simulink model "MODEL_R2021a"  (R2021a)
settings: Solver=FixedStepAuto  StartTime=0.0  StopTime=10.0  FixedStep=0.01  RelTol=1e-3
PreLoadFcn:
  | run('MAIN.m');
undefined symbols (not defined in the file or in its folder): d0, u0, u_tilde
settings Model: OrderedModelArguments=off  Creator=atavo  LastModifiedBy=atavo

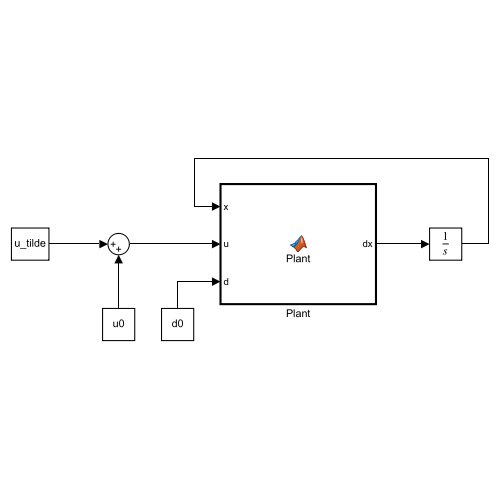
[thumbnail: Simulink's stored preview of the top-level diagram]
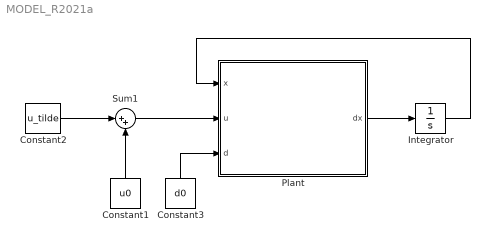
== system MODEL_R2021a ==
  Constant1 : Constant  Value=u0
  Constant2 : Constant  Value=u_tilde
  Constant3 : Constant  Value=d0
  Integrator : Integrator
  Plant : MATLAB Function  TreatAsAtomicUnit=on
  Sum1 : Sum  Inputs=|++
  wires:
  Plant/1(dx) -> Integrator/1
  Integrator/1 -> Plant/1(x)
  Sum1/1 -> Plant/2(u)
  Constant1/1 -> Sum1/2
  Constant2/1 -> Sum1/1
  Constant3/1 -> Plant/3(d)

== matlab function MODEL_R2021a/Plant ==
  data: x input; dx output; u input; d input
function dx = Plant(x,u,d)

    global rho S v0 Cx N_wheels CR
    global g Cy rk r_x r_y r_z m J
    
    g   = 9.81;                         % [m/s^2] gravity acceleration
    rho = 1.225;                        % [kg/m^3] air density
    Cx  = 0.3;                          % drag coefficient 
    Cy  = 0.3;                          % drag coefficient
    rk  = 1;                            % dry asphalt
    v0  = 50/3.6;
    
    r_x = [1.4 1.4 -1.6 -1.6];
    r_y = [0.9 -0.9 0.9 -0.9];
    r_z = 0.70;
    S   = 2.4;                          % [m^2] cross surface
    m   = 1200;                         % [kg] vehicle mass
    J   = m*(r_x(4)^2+r_y(1)^2)^2;      % Vehicle inertia
    
    CR = 0.05;                          % coefficiente attrito resistenza delle ruote

    posin_x     = x(1);
    posin_y     = x(2);
    v_x         = x(3);
    v_y         = x(4);
    omega       = x(5);
    psi         = x(6);

    AeroForce   = 0.5*rho*S *[(v_x^2)*Cx
                              (v_y^2)*Cy];

    mu_body     = zeros(2,4);
    f_x_wheels  = zeros(1,4);
    f_y_wheels  = zeros(1,4);

for i = 1:4

    Rot_btow        = [+cos(delta_w(i)) sin(delta_w(i))
                       -sin(delta_w(i)) cos(delta_w(i))];
    
    V_wheels        = Rot_btow*([-omega*r_y(i) ; omega*r_x(i)] + [v_x ; v_y]);

    beta_wheel      = atan(V_wheels(2)/V_wheels(1));
   
    mu_lambda       = mu_long(rk, lambdas(i));                                 % Dry asphalt
    mu_beta         = mu_long(rk, beta_wheel);                                 % Dry asphalt
    
    mu_body(1,i)    = mu_lambda;
    mu_body(2,i)    = mu_beta;
    
end
    
    N               = m*g;
    
    H               = [ones(1,4)
                        -r_x
                         r_y   ];
    
    N_wheels        = pinv(H) * [         N
                                  0.5*rho*(v_x^2)*S*Cx*r_z
                                          0                ];

for i = 1:4
    f_x_wheels(i) = + N_wheels(i)*mu_body(1,i);
    f_y_wheels(i) = - N_wheels(i)*mu_body(2,i);

    f_x     = f_x + (cos(delta_w(i))*f_x_wheels(i) -sin(delta_w(i))*f_y_wheels(i));
    f_y     = f_y + (sin(delta_w(i))*f_x_wheels(i) +cos(delta_w(i))*f_y_wheels(i));
    tau     = tau + (sin(delta_w(i))*f_y_wheels(i) -cos(delta_w(i))*f_x_wheels(i))*r_y(i) + (sin(delta_w(i))*f_x_wheels(i) +cos(delta_w(i))*f_y_wheels(i))*r_x(i);
end 

dv_x        = (f_x + (m*omega*v_y) - (0.5*rho*S*(v^2)*Cx))/m;
dv_y        = (f_y - (m*omega*v_x))/m;
domega      = tau/J;

dx          = [v_x*cos(psi)
               v_y*sin(psi)
               dv_x
               dv_y
               domega
               omega];                                                      % Derivata degli stati

end

function mu = mu_long(i,lambda) %12.1d

% 1) Dry asphalt
% 2) wet asphalt
% 3) Snow
% 4) Ice
% 5) Dry Cobblestone
% 6) wet cobblestone
theta1 = [1.28 0.86 0.19 0.05 1.37 0.4];
theta2 = [23.99 33.82 94.13 306.39 6.46 33.71];
theta3 = [0.52 0.35 0.05 0 0.67 0.12];

mu = sign(lambda).*theta1(i).*(1-exp(-abs(lambda)*theta2(i)))-theta3(i)*lambda;
end
